simulink library "asbhl20sensors"  (R2016b)
settings: Solver=VariableStepAuto  StartTime=0.0  StopTime=10.0  RelTol=1e-3
Description:
  | HL-20 vehicle flight parameter sensors component module (stub)
settings Model: Creator=The MathWorks, Inc.  LastModifiedBy=The MathWorks, Inc.
settings DataIOCC: SaveFormat=Array  SignalLoggingSaveFormat=ModelDataLogs
settings OptimizationCC: BlockReduction=off  BooleanDataType=off
settings DebuggingCC: SaveWithParameterizedLinksMsg=none  UnderspecifiedInitializationDetection=Classic  MergeDetectMultiDrivingBlocksExec=none  SignalResolutionControl=TryResolveAllWithWarning  MultiTaskCondExecSysMsg=none  StrictBusMsg=None
settings HardwareCC: ProdBitPerPointer=32  ProdBitPerSizeT=32  ProdBitPerPtrDiffT=32  ProdLargestAtomicFloat=None  ProdIntDivRoundTo=Undefined  ProdEndianess=Unspecified  ProdWordSize=32  ProdHWDeviceType=32-bit Generic  TargetUnknown=on
settings ModelReferenceCC: PropagateSignalLabelsOutOfModel=off
settings ConfigComp: CovMetricSettings=dw  CovHtmlReporting=on  CovSaveCumulativeToWorkspaceVar=on  CovSaveSingleToWorkspaceVar=on  CovExternalEMLEnable=off

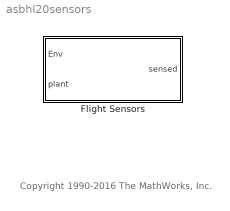
== system asbhl20sensors ==
  note: Copyright 1990-2016 The MathWorks, Inc.
  Flight Sensors : Subsystem

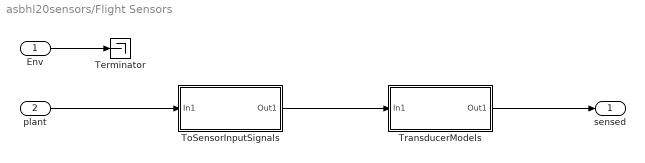
== system asbhl20sensors/Flight Sensors ==
  Env : Inport
  plant : Inport  Port=2
  Terminator : Terminator
  ToSensorInputSignals : Subsystem
  TransducerModels : Subsystem
  sensed : Outport
  wires:
  plant/1 -> ToSensorInputSignals/1(In1)
  TransducerModels/1(Out1) -> sensed/1
  Env/1 -> Terminator/1
  ToSensorInputSignals/1(Out1) -> TransducerModels/1(In1)

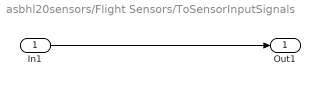
== system asbhl20sensors/Flight Sensors/ToSensorInputSignals ==
  In1 : Inport
  Out1 : Outport
  wires:
  In1/1 -> Out1/1

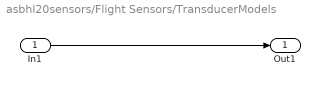
== system asbhl20sensors/Flight Sensors/TransducerModels ==
  In1 : Inport
  Out1 : Outport
  wires:
  In1/1 -> Out1/1
